simulink model "system"  (R2021a)
settings: Solver=VariableStepAuto  StartTime=0.0  StopTime=10.0  RelTol=1e-3
settings Model: Creator=Nikitos  LastModifiedBy=Nikitos

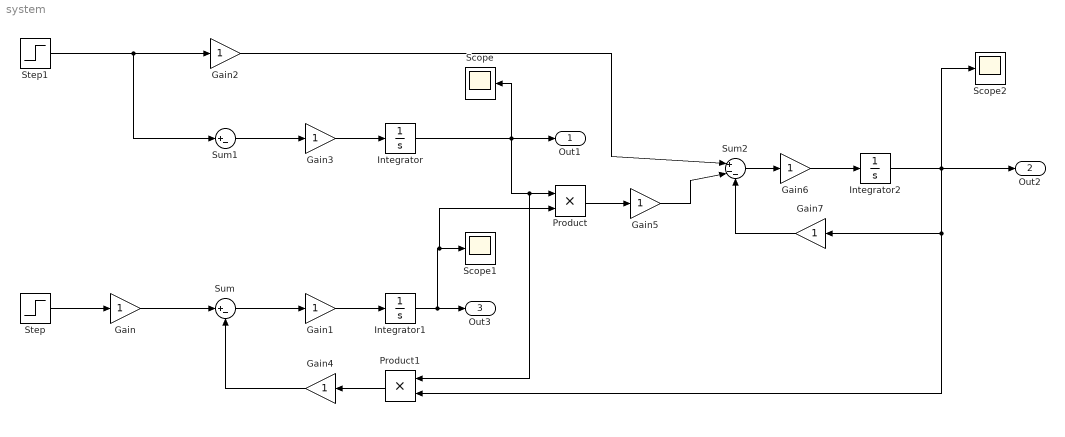
== system system ==
  Gain{,1..7} (8 alike) : Gain
  Integrator : Integrator
  Integrator1 : Integrator
  Integrator2 : Integrator
  Product : Product
  Product1 : Product
  Scope : Scope
  Scope1 : Scope
  Scope2 : Scope
  Step : Step  SampleTime=0
  Step1 : Step  SampleTime=0
  Sum : Sum  Inputs=|+-
  Sum1 : Sum  Inputs=|+-
  Sum2 : Sum  Inputs=|+--
  Out1 : Outport
  Out2 : Outport  Port=2
  Out3 : Outport  Port=3
  wires:
  Step/1 -> Gain/1
  Gain/1 -> Sum/1
  Sum/1 -> Gain1/1
  Step1/1 -> Sum1/1, Gain2/1
  Sum1/1 -> Gain3/1
  Gain3/1 -> Integrator/1
  Gain1/1 -> Integrator1/1
  Gain4/1 -> Sum/2
  Product1/1 -> Gain4/1
  Integrator1/1 -> Product/2, Scope1/1, Out3/1
  Integrator/1 -> Out1/1, Scope/1, Product/1, Product1/1
  Gain5/1 -> Sum2/2
  Gain2/1 -> Sum2/1
  Product/1 -> Gain5/1
  Sum2/1 -> Gain6/1
  Gain6/1 -> Integrator2/1
  Integrator2/1 -> Product1/2, Gain7/1, Scope2/1, Out2/1
  Gain7/1 -> Sum2/3
